simulink model "W11_City_Highway_cs"  (R2019a)
settings: Solver=ode5  StartTime=0.0  StopTime=529  FixedStep=1/1  RelTol=1e-3
PreLoadFcn:
  | mbxruntime.callbacks.PreLoadFcn(bdroot);
PostLoadFcn:
  | mbxruntime.callbacks.PostLoadFcn(bdroot);
InitFcn:
  | mbxruntime.callbacks.InitFcn(bdroot);
StartFcn:
  | mbxruntime.callbacks.StartFcn(bdroot);
StopFcn:
  | mbxruntime.callbacks.StopFcn(bdroot);
model workspace: external: MAT-File .\W11_city_highway_cs_hws.mat (data not in the file)
undefined symbols (not defined in the file or in its folder): InitImageOutputDir, W11_city_highway_cs_05e81c5221fce2b9, W11_city_highway_cs_BMW_X5_SUV_2_Path_pathUniqueID
(part 2 of 2)

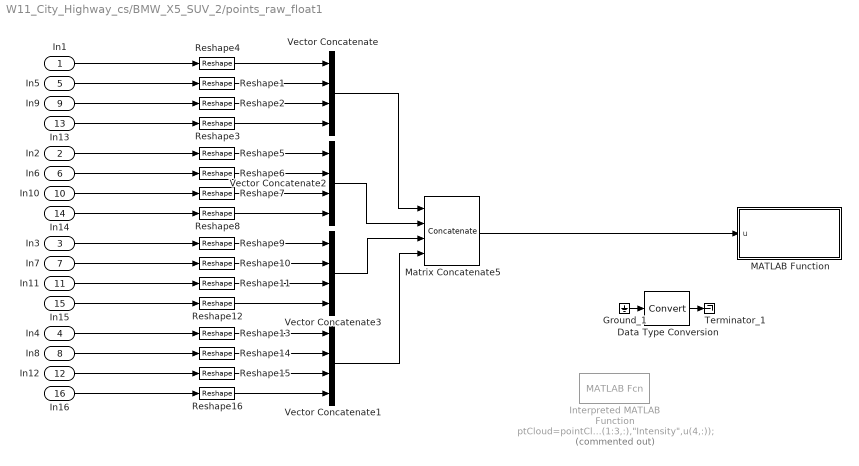
== system W11_City_Highway_cs/BMW_X5_SUV_2/points_raw_float1 ==
  In1 : Inport
  In2 : Inport  Port=2
  In3 : Inport  Port=3
  In4 : Inport  Port=4
  In5 : Inport  Port=5
  In6 : Inport  Port=6
  In7 : Inport  Port=7
  In8 : Inport  Port=8
  In9 : Inport  Port=9
  In10 : Inport  Port=10
  In11 : Inport  Port=11
  In12 : Inport  Port=12
  In13 : Inport  Port=13
  In14 : Inport  Port=14
  In15 : Inport  Port=15
  In16 : Inport  Port=16
  Data Type Conversion : DataTypeConversion
  Ground_1 : Ground
  Interpreted MATLAB Function : MATLABFcn  Commented=on  MATLABFcn="ptCloud=pointCloud(u(1:3,:),\"Intensity\",u(4,:));"
  MATLAB Function : MATLAB Function  TreatAsAtomicUnit=on
  Matrix Concatenate5 : Concatenate  NumInputs=4  Mode=Multidimensional array  ConcatenateDimension=2
  Reshape{1..16} (16 alike) : Reshape
  Terminator_1 : Terminator
  Vector Concatenate{,1..3} (4 alike) : Concatenate  NumInputs=4
  wires:
  In1/1 -> Reshape4/1
  In2/1 -> Reshape5/1
  In3/1 -> Reshape9/1
  In4/1 -> Reshape13/1
  In5/1 -> Reshape1/1
  In6/1 -> Reshape6/1
  In7/1 -> Reshape10/1
  In8/1 -> Reshape14/1
  In9/1 -> Reshape2/1
  In10/1 -> Reshape7/1
  In11/1 -> Reshape11/1
  In12/1 -> Reshape15/1
  In13/1 -> Reshape3/1
  In14/1 -> Reshape8/1
  In15/1 -> Reshape12/1
  In16/1 -> Reshape16/1
  Reshape4/1 -> Vector Concatenate/1
  Reshape1/1 -> Vector Concatenate/2
  Reshape2/1 -> Vector Concatenate/3
  Reshape3/1 -> Vector Concatenate/4
  Reshape5/1 -> Vector Concatenate2/1
  Reshape6/1 -> Vector Concatenate2/2
  Reshape7/1 -> Vector Concatenate2/3
  Reshape8/1 -> Vector Concatenate2/4
  Reshape9/1 -> Vector Concatenate3/1
  Reshape10/1 -> Vector Concatenate3/2
  Reshape11/1 -> Vector Concatenate3/3
  Reshape12/1 -> Vector Concatenate3/4
  Reshape13/1 -> Vector Concatenate1/1
  Reshape14/1 -> Vector Concatenate1/2
  Reshape15/1 -> Vector Concatenate1/3
  Reshape16/1 -> Vector Concatenate1/4
  Vector Concatenate/1 -> Matrix Concatenate5/1
  Vector Concatenate2/1 -> Matrix Concatenate5/2
  Vector Concatenate3/1 -> Matrix Concatenate5/3
  Vector Concatenate1/1 -> Matrix Concatenate5/4
  Matrix Concatenate5/1 -> MATLAB Function/1(u)
  Ground_1/1 -> Data Type Conversion/1
  Data Type Conversion/1 -> Terminator_1/1

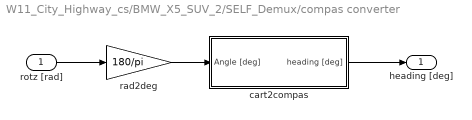
== system W11_City_Highway_cs/BMW_X5_SUV_2/SELF_Demux/compas converter ==
  rotz [rad] : Inport
  cart2compas : Subsystem
  rad2deg : Gain  Gain=180/pi
  heading [deg] : Outport
  wires:
  rad2deg/1 -> cart2compas/1(Angle [deg])
  rotz [rad]/1 -> rad2deg/1
  cart2compas/1(heading [deg]) -> heading [deg]/1

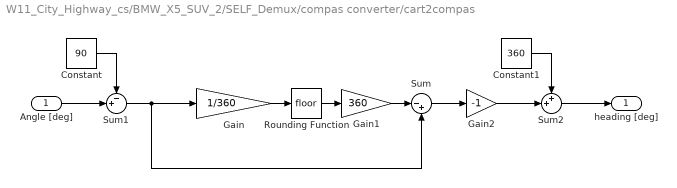
== system W11_City_Highway_cs/BMW_X5_SUV_2/SELF_Demux/compas converter/cart2compas ==
  Angle [deg] : Inport
  Constant : Constant  Value=90
  Constant1 : Constant  Value=360
  Gain : Gain  Gain=1/360
  Gain1 : Gain  Gain=360
  Gain2 : Gain  Gain=-1
  Rounding Function : Rounding
  Sum : Sum  Inputs=|-+
  Sum1 : Sum  Inputs=-+|
  Sum2 : Sum  Inputs=++|
  heading [deg] : Outport
  wires:
  Gain/1 -> Rounding Function/1
  Rounding Function/1 -> Gain1/1
  Gain1/1 -> Sum/1
  Angle [deg]/1 -> Sum1/2
  Sum/1 -> Gain2/1
  Sum1/1 -> Gain/1, Sum/2
  Constant/1 -> Sum1/1
  Gain2/1 -> Sum2/2
  Constant1/1 -> Sum2/1
  Sum2/1 -> heading [deg]/1

== matlab function W11_City_Highway_cs/BMW_X5_SUV_2/points_raw_float1/MATLAB Function ==
  data: u input

function fcn(u)
Path_to_Data_Folder = "..\Pointcloud_Files\";
coder.extrinsic('clock')
coder.extrinsic('num2str')
coder.extrinsic('strcat')
coder.extrinsic('pcwrite')
coder.extrinsic('pointCloud')
xyzPoints=u(:,1:3);
Intensities=u(:,4);
ptCloud=pointCloud(xyzPoints,"Intensity",Intensities);

c=clock;
filename=strcat(Path_to_Data_Folder,"pcd",num2str(fix(c(4))),num2str(fix(c(5))),num2str(fix(1000*c(6))),".pcd");
pcwrite(ptCloud,filename);
